simulink model "mOneLossMap"  (R2021b)
settings: Solver=VariableStepAuto  StartTime=0.0  StopTime=10.0  RelTol=1e-3
values from neighbouring files (symbols this model uses):
  speedVal = SpeedMat(end,end)    [tLossMaps.m]    (also in tLossMapsWithDCV.m = SpeedVec(end))
  torqueVal = ShaftTorqueMat(end,end)    [tLossMaps.m]    (also in tLossMapsWithDCV.m = TorqueVec(end))
  xVec = linspace(xMin, xMax, xLen)    [tLossMaps.m]    (also in tLossMapsWithDCV.m = linspace(min(xMat(:)), max(xMat(:)), nx))
  yVec = linspace(yMin, yMax, yLen)    [tLossMaps.m]    (also in tLossMapsWithDCV.m = linspace(min(yMat(:)), max(yMat(:)), ny))
  zgMat = zInterpolant(xgrid, ygrid)    [tLossMaps.m]
settings Model: Creator=agonzale  LastModifiedBy=agonzale

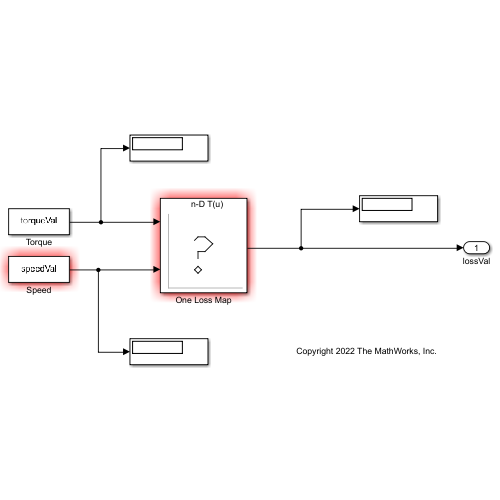
[thumbnail: Simulink's stored preview of the top-level diagram]
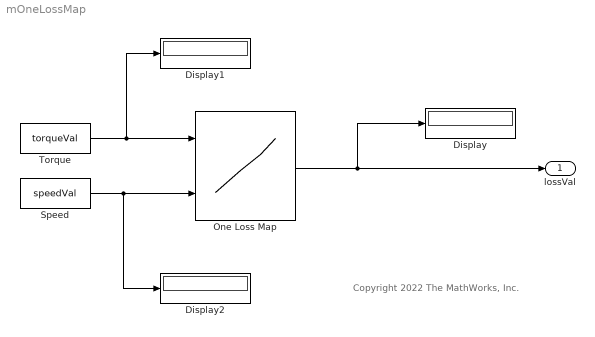
== system mOneLossMap ==
  note: Copyright 2022 The MathWorks, Inc.
  Display : Display
  Display1 : Display
  Display2 : Display
  One Loss Map : Lookup_n-D  BreakpointsForDimension1=xVec  BreakpointsForDimension2=yVec  Table=zgMat  ExtrapMethod=Clip  UseLastTableValue=on  InternalRulePriority=Speed  RndMeth=Simplest  InputSameDT=on
      settings: InputPortMap=u0,u1
  Speed : Constant  Value=speedVal
  Torque : Constant  Value=torqueVal
  lossVal : Outport
  wires:
  Torque/1 -> Display1/1, One Loss Map/1
  Speed/1 -> Display2/1, One Loss Map/2
  One Loss Map/1 -> Display/1, lossVal/1
